simulink model "ModelCurrentState"  (R2024b)
settings: Solver=VariableStepAuto  StartTime=0.0  StopTime=StopTime  MaxStep=0.001  RelTol=1e-3
model workspace: external: MAT-File 3DModelInputs.mat (data not in the file)
undefined symbols (not defined in the file): GripStrength, KillswitchFinalValue, KillswitchInitialValue, KillswitchStepTime, LeftLowerArmLength, PlaneTilt, RightLowerArmLength, UpperTorsoLength, X, Y, Z
libraries: nesl_utility x408, sm_lib x139, matrix_library x11, simulink x1
(part 12 of 14)

== matlab function ModelCurrentState/LW Input Function/Left Wrist Torque ==
  data: Time input; Killswitch input; JointTorqueLWX output; LWInputXA parameter; LWInputYA parameter; LWInputXB parameter; LWInputYB parameter; LWPositionSetpointX parameter; GlobalGain parameter; JointTorqueLWY output; LWConstantX parameter; LWConstantY parameter; LWTimeGainX parameter; LWTimeGainY parameter; LWInputXC parameter; LWInputYC parameter; LWPositionGainX parameter; LWPositionGainY parameter; TargetLWPositionX parameter; ModelingMode parameter; GlobalPCGain parameter; GlobalVCGain parameter; DampeningGlobalGain parameter; TargetImpactTime parameter; KinematicMode parameter; LWPositionSetpointY parameter; LWStartPositionX parameter; LWStartPositionY parameter; LWStartVelocityX parameter; LWStartVelocityY parameter; LWVCGainX parameter; LWVCGainY parameter; LWPCGainX parameter; LWPCGainY parameter; LWPositionInputX output; LWPositionInputY output; LWVelocityInputX output; LWVelocityInputY output; LWAccelerationInputX output; LWAccelerationInputY output; ZVCFLWTorqueX parameter; ZVCFLWTorqueY parameter; LWAoX parameter; LWAoY parameter; LWDampeningX parameter; LWDampeningY parameter; TargetLWPositionY parameter; TargetLWVelocityX parameter; TargetLWVelocityY parameter; LWPositionX input; LWPositionY input; LWVelocityX input; LWVelocityY input; LWAfX parameter; LWAfY parameter; LWInputXD parameter; LWInputXE parameter; LWInputXF parameter; LWInputXG parameter; LWInputYD parameter; LWInputYE parameter; LWInputYF parameter; LWInputYG parameter; LWLocaltoGlobalR input; LWTorqueGlobal input; LWJointTorqueInputGlobal output; LWConstraintTorque output
function [JointTorqueLWX,JointTorqueLWY,LWPositionInputX, LWPositionInputY,...
    LWVelocityInputX,LWVelocityInputY,LWAccelerationInputX,LWAccelerationInputY,...
    LWJointTorqueInputGlobal,LWConstraintTorque]...
    = fcn(Time,Killswitch, LWInputXA,LWInputYA, LWInputXB,LWInputYB, LWPositionSetpointX,GlobalGain,...
    LWConstantX, LWConstantY, LWTimeGainX, LWTimeGainY,...
    LWInputXC, LWInputYC, LWPositionGainX, LWPositionGainY,...
    TargetLWPositionX, ModelingMode,GlobalPCGain, GlobalVCGain,DampeningGlobalGain,TargetImpactTime,KinematicMode, LWPositionSetpointY, LWStartPositionX,...
    LWStartPositionY, LWStartVelocityX, LWStartVelocityY, LWVCGainX,...
    LWVCGainY, LWPCGainX, LWPCGainY, ZVCFLWTorqueX, ZVCFLWTorqueY, LWAoX,...
    LWAoY, LWDampeningX, LWDampeningY, TargetLWPositionY, TargetLWVelocityX,...
    TargetLWVelocityY, LWPositionX, LWPositionY, LWVelocityX, LWVelocityY,...
    LWAfX, LWAfY,LWInputXD, LWInputXE, LWInputXF, LWInputXG, LWInputYD, LWInputYE, LWInputYF, LWInputYG,LWLocaltoGlobalR,LWTorqueGlobal)

%Tau=Time/TargetImpactTime;
t=Time;

% %%%%%%%%%%%%%%%%%%%%%%%%%%%%%%%%%%%%%%%%%%%
% % Kinetic Input Selection and Calculation
% %%%%%%%%%%%%%%%%%%%%%%%%%%%%%%%%%%%%%%%%%%%

if ModelingMode==0
    % Values are all set to zero.
    JointTorqueLWX=0;
    JointTorqueLWY=0;
elseif ModelingMode==1
    % Control based strategy. Values are based on difference in value
    % between the current state and desired state.
    % LW Joint Rotational Deltas
    DeltaLWPositionX=LWPositionX-TargetLWPositionX;
    DeltaLWPositionY=LWPositionY-TargetLWPositionY;
    DeltaLWVelocityX=LWVelocityX-TargetLWVelocityX;
    DeltaLWVelocityY=LWVelocityY-TargetLWVelocityY;
    % Control Based Strategy
    JointTorqueLWX=DeltaLWPositionX*LWPCGainX*GlobalPCGain-DeltaLWVelocityX*LWVCGainX*GlobalVCGain-DampeningGlobalGain*LWDampeningX*LWVelocityX;
    JointTorqueLWY=DeltaLWPositionY*LWPCGainY*GlobalPCGain-DeltaLWVelocityY*LWVCGainY*GlobalVCGain-DampeningGlobalGain*LWDampeningY*LWVelocityY;
elseif ModelingMode==2
    % Forward Dynamics Based Strategy. Values are computed based on a
    % polynomial and a combination of dampening and position gained
    % factors.
    JointTorqueLWX=Killswitch*GlobalGain*(LWConstantX+LWTimeGainX*Time-LWPositionGainX*(LWPositionX-LWPositionSetpointX)...
    -LWDampeningX*LWVelocityX);
    JointTorqueLWY=Killswitch*GlobalGain*(LWConstantY+LWTimeGainY*Time-LWPositionGainY*(LWPositionY-LWPositionSetpointY)...
    -LWDampeningY*LWVelocityY);
elseif ModelingMode==3
    JointTorqueLWX=HexPolyInputFunction(LWInputXA,LWInputXB,LWInputXC,LWInputXD,LWInputXE,LWInputXF,LWInputXG,Time)*Killswitch;
    JointTorqueLWY=HexPolyInputFunction(LWInputYA,LWInputYB,LWInputYC,LWInputYD,LWInputYE,LWInputYF,LWInputYG,Time)*Killswitch;  
else
    %ZVCF Based Joint Torques. Values are pulled from model workspace and
    %held constant.
    JointTorqueLWX=ZVCFLWTorqueX;
    JointTorqueLWY=ZVCFLWTorqueY;
end

% Create a global vector of the joint torque inputs
LWJointTorqueInputLocal=cat(1,JointTorqueLWX,JointTorqueLWY,0);
LWJointTorqueInputGlobal=LWLocaltoGlobalR*LWJointTorqueInputLocal;
% 
% Compare total torque measured to input torques applied to see the
% constraint torque
LWConstraintTorque=LWTorqueGlobal-LWJointTorqueInputGlobal;

% %%%%%%%%%%%%%%%%%%%%%%%%%%%%%%%%%%%%%%%%%%%
% % Kinematic Input Selection and Calculation
% %%%%%%%%%%%%%%%%%%%%%%%%%%%%%%%%%%%%%%%%%%%

if KinematicMode==0
    % All kinematic values set to zero.
    LWPositionInputX=0;
    LWPositionInputY=0;
    LWVelocityInputX=0;
    LWVelocityInputY=0;
    LWAccelerationInputX=0;
    LWAccelerationInputY=0;
elseif KinematicMode==1
    % 1st Order Acceleration, 2nd Order Velocity, 3rd Order Position Solution
    PTX=TargetLWPositionX;       
    VTX=TargetLWVelocityX;
    PTY=TargetLWPositionY;
    VTY=TargetLWVelocityY;
    % Define Starting Position and Velocity
    PIX=LWStartPositionX;
    VIX=LWStartVelocityX;
    PIY=LWStartPositionY;
    VIY=LWStartVelocityY;
    AX=3*((VTX+VIX)*TargetImpactTime-2*(PTX-PIX))/TargetImpactTime^3;         % Constant in position equation
    BX=-2*((VTX+2*VIX)*TargetImpactTime-3*(PTX-PIX))/TargetImpactTime^2;         % Constant in position equation
    CX=VIX;         % Starting Velocity at Time Zero
    DX=PIX;         % Starting Position at Time Zero
    AY=3*((VTY+VIY)*TargetImpactTime-2*(PTY-PIY))/TargetImpactTime^3;         % Constant in position equation
    BY=-2*((VTY+2*VIY)*TargetImpactTime-3*(PTY-PIY))/TargetImpactTime^2;         % Constant in position equation
    CY=VIY;         % Starting Velocity at Time Zero
    DY=PIY;         % Starting Position at Time Zero
    % Equation for position as a function of time
    LWPositionInputX=AX*Time^3/3+BX*Time^2/2+CX*Time+DX;
    LWPositionInputY=AY*Time^3/3+BY*Time^2/2+CY*Time+DY;
    LWVelocityInputX=AX*Time^2+BX*Time+CX;
    LWVelocityInputY=AY*Time^2+BY*Time+CY;
    LWAccelerationInputX=2*AX*Time+BX;
    LWAccelerationInputY=2*AY*Time+BY;
elseif KinematicMode==2
    % 2nd Order Acceleration, 3rd Order Velocity, 4th Order Position Solution
    Tt=TargetImpactTime;
    t=Time;
    PoX=LWStartPositionX;
    PoY=LWStartPositionY;
    VoX=LWStartVelocityX;
    VoY=LWStartVelocityY;
    PfX=TargetLWPositionX;
    PfY=TargetLWPositionY;
    VfX=TargetLWVelocityX;
    VfY=TargetLWVelocityY;
    AoX=LWAoX;
    AoY=LWAoY;
    LWPositionInputX=PoX + VoX*t + (AoX*t^2)/2 - (t^3*(4*PoX - 4*PfX + Tt*VfX + 3*Tt*VoX + AoX*Tt^2))/Tt^3 + (t^4*(6*PoX - 6*PfX + 2*Tt*VfX + 4*Tt*VoX + AoX*Tt^2))/(2*Tt^4);
    LWPositionInputY=PoY + VoY*t + (AoY*t^2)/2 - (t^3*(4*PoY - 4*PfY + Tt*VfY + 3*Tt*VoY + AoY*Tt^2))/Tt^3 + (t^4*(6*PoY - 6*PfY + 2*Tt*VfY + 4*Tt*VoY + AoY*Tt^2))/(2*Tt^4);
    LWVelocityInputX=VoX + AoX*t - (3*t^2*(4*PoX - 4*PfX + Tt*VfX + 3*Tt*VoX + AoX*Tt^2))/Tt^3 + (2*t^3*(6*PoX - 6*PfX + 2*Tt*VfX + 4*Tt*VoX + AoX*Tt^2))/Tt^4;
    LWVelocityInputY=VoY + AoY*t - (3*t^2*(4*PoY - 4*PfY + Tt*VfY + 3*Tt*VoY + AoY*Tt^2))/Tt^3 + (2*t^3*(6*PoY - 6*PfY + 2*Tt*VfY + 4*Tt*VoY + AoY*Tt^2))/Tt^4;
    LWAccelerationInputX=AoX + (6*t^2*(6*PoX - 6*PfX + 2*Tt*VfX + 4*Tt*VoX + AoX*Tt^2))/Tt^4 - (6*t*(4*PoX - 4*PfX + Tt*VfX + 3*Tt*VoX + AoX*Tt^2))/Tt^3;
    LWAccelerationInputY=AoY + (6*t^2*(6*PoY - 6*PfY + 2*Tt*VfY + 4*Tt*VoY + AoY*Tt^2))/Tt^4 - (6*t*(4*PoY - 4*PfY + Tt*VfY + 3*Tt*VoY + AoY*Tt^2))/Tt^3;
else
    % 3rd Order Acceleration, 4th Order Velocity, 5th Order Position Solution
    Tt=TargetImpactTime;
    t=Time;
    PoX=LWStartPositionX;
    PoY=LWStartPositionY;
    VoX=LWStartVelocityX;
    VoY=LWStartVelocityY;
    PfX=TargetLWPositionX;
    PfY=TargetLWPositionY;
    VfX=TargetLWVelocityX;
    VfY=TargetLWVelocityY;
    AoX=LWAoX;
    AoY=LWAoY;
    AfX=LWAfX;
    AfY=LWAfY;
    LWPositionInputX=PoX+VoX*t+(AoX*t^2)/2-(t^5*(12*PoX-12*PfX+6*Tt*VfX+6*Tt*VoX-AfX*Tt^2+AoX*Tt^2))/(2*Tt^5)-(t^3*(20*PoX-20*PfX+8*Tt*VfX+12*Tt*VoX-AfX*Tt^2+3*AoX*Tt^2))/(2*Tt^3)+(t^4*(30*PoX-30*PfX+14*Tt*VfX+16*Tt*VoX-2*AfX*Tt^2+3*AoX*Tt^2))/(2*Tt^4);
    LWPositionInputY=PoY+VoY*t+(AoY*t^2)/2-(t^5*(12*PoY-12*PfY+6*Tt*VfY+6*Tt*VoY-AfY*Tt^2+AoY*Tt^2))/(2*Tt^5)-(t^3*(20*PoY-20*PfY+8*Tt*VfY+12*Tt*VoY-AfY*Tt^2+3*AoY*Tt^2))/(2*Tt^3)+(t^4*(30*PoY-30*PfY+14*Tt*VfY+16*Tt*VoY-2*AfY*Tt^2+3*AoY*Tt^2))/(2*Tt^4);  
    LWVelocityInputX=VoX+AoX*t-(5*t^4*(12*PoX-12*PfX+6*Tt*VfX+6*Tt*VoX-AfX*Tt^2+AoX*Tt^2))/(2*Tt^5)-(3*t^2*(20*PoX-20*PfX+8*Tt*VfX+12*Tt*VoX-AfX*Tt^2+3*AoX*Tt^2))/(2*Tt^3)+(2*t^3*(30*PoX-30*PfX+14*Tt*VfX+16*Tt*VoX-2*AfX*Tt^2+3*AoX*Tt^2))/Tt^4;
    LWVelocityInputY=VoY+AoY*t-(5*t^4*(12*PoY-12*PfY+6*Tt*VfY+6*Tt*VoY-AfY*Tt^2+AoY*Tt^2))/(2*Tt^5)-(3*t^2*(20*PoY-20*PfY+8*Tt*VfY+12*Tt*VoY-AfY*Tt^2+3*AoY*Tt^2))/(2*Tt^3)+(2*t^3*(30*PoY-30*PfY+14*Tt*VfY+16*Tt*VoY-2*AfY*Tt^2+3*AoY*Tt^2))/Tt^4;
    LWAccelerationInputX=AoX-(3*t*(20*PoX-20*PfX+8*Tt*VfX+12*Tt*VoX-AfX*Tt^2+3*AoX*Tt^2))/Tt^3-(10*t^3*(12*PoX-12*PfX+6*Tt*VfX+6*Tt*VoX-AfX*Tt^2+AoX*Tt^2))/Tt^5+(6*t^2*(30*PoX-30*PfX+14*Tt*VfX+16*Tt*VoX-2*AfX*Tt^2+3*AoX*Tt^2))/Tt^4;
    LWAccelerationInputY=AoY-(3*t*(20*PoY-20*PfY+8*Tt*VfY+12*Tt*VoY-AfY*Tt^2+3*AoY*Tt^2))/Tt^3-(10*t^3*(12*PoY-12*PfY+6*Tt*VfY+6*Tt*VoY-AfY*Tt^2+AoY*Tt^2))/Tt^5+(6*t^2*(30*PoY-30*PfY+14*Tt*VfY+16*Tt*VoY-2*AfY*Tt^2+3*AoY*Tt^2))/Tt^4;
end


% Calculate Higher Order Derivatives of the Position Outputs
LWJerkX=gradient(LWAccelerationInputX,t);
LWJerkY=gradient(LWAccelerationInputY,t);
LWSnapX=gradient(LWJerkX,t);
LWSnapY=gradient(LWJerkY,t);
LWCrackleX=gradient(LWSnapX,t);
LWCrackleY=gradient(LWSnapY,t);
LWPopX=gradient(LWCrackleX,t);
LWPopY=gradient(LWCrackleY,t);

== matlab function ModelCurrentState/RW Input Function/Right Wrist Torque ==
  data: Time input; Killswitch input; JointTorqueRWX output; RWInputXA parameter; RWInputYA parameter; RWInputXB parameter; RWInputYB parameter; RWPositionSetpointX parameter; GlobalGain parameter; JointTorqueRWY output; RWConstantX parameter; RWConstantY parameter; RWTimeGainX parameter; RWTimeGainY parameter; RWInputXC parameter; RWInputYC parameter; RWPositionGainX parameter; RWPositionGainY parameter; TargetRWPositionX parameter; ModelingMode parameter; GlobalPCGain parameter; GlobalVCGain parameter; DampeningGlobalGain parameter; TargetImpactTime parameter; KinematicMode parameter; RWVCGainY parameter; RWPCGainX parameter; RWPCGainY parameter; ZVCFRWTorqueX parameter; ZVCFRWTorqueY parameter; TargetRWPositionY parameter; TargetRWVelocityX parameter; TargetRWVelocityY parameter; RWAoX parameter; RWPositionInputX output; RWPositionInputY output; RWVelocityInputX output; RWVelocityInputY output; RWAccelerationInputX output; RWAccelerationInputY output; RWAoY parameter; RWDampeningX parameter; RWDampeningY parameter; RWPositionX input; RWPositionY input; RWStartPositionX parameter; RWStartPositionY parameter; RWStartVelocityX parameter; RWStartVelocityY parameter; RWVCGainX parameter; RWPositionSetpointY parameter; RWVelocityX input; RWVelocityY input; RWAfX parameter; RWAfY parameter; RWInputXD parameter; RWInputXE parameter; RWInputXF parameter; RWInputXG parameter; RWInputYD parameter; RWInputYE parameter; RWInputYF parameter; RWInputYG parameter; RWLocaltoGlobalR input; RWTorqueGlobal input; RWJointTorqueInputGlobal output; RWConstraintTorque output
function [JointTorqueRWX,JointTorqueRWY,RWPositionInputX, RWPositionInputY,...
    RWVelocityInputX,RWVelocityInputY,RWAccelerationInputX,RWAccelerationInputY,...
    RWJointTorqueInputGlobal,RWConstraintTorque]...
    = fcn(Time,Killswitch, RWInputXA,RWInputYA, RWInputXB,RWInputYB, RWPositionSetpointX,GlobalGain,...
    RWConstantX, RWConstantY, RWTimeGainX, RWTimeGainY,...
    RWInputXC, RWInputYC, RWPositionGainX, RWPositionGainY,...
    TargetRWPositionX, ModelingMode,GlobalPCGain, GlobalVCGain,...
    DampeningGlobalGain,TargetImpactTime,KinematicMode, RWVCGainY,...
    RWPCGainX, RWPCGainY, ZVCFRWTorqueX, ...
    ZVCFRWTorqueY, TargetRWPositionY, TargetRWVelocityX, TargetRWVelocityY,...
    RWAoX, RWAoY, RWDampeningX, RWDampeningY, RWPositionX, RWPositionY, RWStartPositionX,...
    RWStartPositionY, RWStartVelocityX, RWStartVelocityY, RWVCGainX,...
    RWPositionSetpointY, RWVelocityX, RWVelocityY,RWAfX, RWAfY,RWInputXD, RWInputXE, RWInputXF,...
RWInputXG, RWInputYD, RWInputYE, RWInputYF, RWInputYG,RWLocaltoGlobalR,RWTorqueGlobal)

%Tau=Time/TargetImpactTime;
t=Time;

% %%%%%%%%%%%%%%%%%%%%%%%%%%%%%%%%%%%%%%%%%%%
% % Kinetic Input Selection and Calculation
% %%%%%%%%%%%%%%%%%%%%%%%%%%%%%%%%%%%%%%%%%%%

if ModelingMode==0
    % Values are all set to zero.
    JointTorqueRWX=0;
    JointTorqueRWY=0;
elseif ModelingMode==1
    % Control based strategy. Values are based on difference in value
    % between the current state and desired state.
    % RW Joint Rotational Deltas
    DeltaRWPositionX=RWPositionX-TargetRWPositionX;
    DeltaRWPositionY=RWPositionY-TargetRWPositionY;
    DeltaRWVelocityX=RWVelocityX-TargetRWVelocityX;
    DeltaRWVelocityY=RWVelocityY-TargetRWVelocityY;
    % Control Based Strategy
    JointTorqueRWX=DeltaRWPositionX*RWPCGainX*GlobalPCGain-DeltaRWVelocityX*RWVCGainX*GlobalVCGain-DampeningGlobalGain*RWDampeningX*RWVelocityX;
    JointTorqueRWY=DeltaRWPositionY*RWPCGainY*GlobalPCGain-DeltaRWVelocityY*RWVCGainY*GlobalVCGain-DampeningGlobalGain*RWDampeningY*RWVelocityY;
elseif ModelingMode==2
    % Forward Dynamics Based Strategy. Values are computed based on a
    % polynomial and a combination of dampening and position gained
    % factors.
    JointTorqueRWX=Killswitch*GlobalGain*(RWConstantX+RWTimeGainX*Time-RWPositionGainX*(RWPositionX-RWPositionSetpointX)...
    -RWDampeningX*RWVelocityX);
    JointTorqueRWY=Killswitch*GlobalGain*(RWConstantY+RWTimeGainY*Time-RWPositionGainY*(RWPositionY-RWPositionSetpointY)...
    -RWDampeningY*RWVelocityY);
elseif ModelingMode==3
    JointTorqueRWX=HexPolyInputFunction(RWInputXA,RWInputXB,RWInputXC,RWInputXD,RWInputXE,RWInputXF,RWInputXG,Time)*Killswitch;
    JointTorqueRWY=HexPolyInputFunction(RWInputYA,RWInputYB,RWInputYC,RWInputYD,RWInputYE,RWInputYF,RWInputYG,Time)*Killswitch;  
else
    %ZVCF Based Joint Torques. Values are pulled from model workspace and
    %held constant.
    JointTorqueRWX=ZVCFRWTorqueX;
    JointTorqueRWY=ZVCFRWTorqueY;
end

% Create a global vector of the joint torque inputs
RWJointTorqueInputLocal=cat(1,JointTorqueRWX,JointTorqueRWY,0);
RWJointTorqueInputGlobal=RWLocaltoGlobalR*RWJointTorqueInputLocal;

% Compare total torque measured to input torques applied to see the
% constraint torque

RWConstraintTorque=RWTorqueGlobal-RWJointTorqueInputGlobal;

% %%%%%%%%%%%%%%%%%%%%%%%%%%%%%%%%%%%%%%%%%%%
% % Kinematic Input Selection and Calculation
% %%%%%%%%%%%%%%%%%%%%%%%%%%%%%%%%%%%%%%%%%%%

if KinematicMode==0
    % All kinematic values set to zero.
    RWPositionInputX=0;
    RWPositionInputY=0;
    RWVelocityInputX=0;
    RWVelocityInputY=0;
    RWAccelerationInputX=0;
    RWAccelerationInputY=0;
elseif KinematicMode==1
    % 1st Order Acceleration, 2nd Order Velocity, 3rd Order Position Solution
    PTX=TargetRWPositionX;       
    VTX=TargetRWVelocityX;
    PTY=TargetRWPositionY;
    VTY=TargetRWVelocityY;
    % Define Starting Position and Velocity
    PIX=RWStartPositionX;
    VIX=RWStartVelocityX;
    PIY=RWStartPositionY;
    VIY=RWStartVelocityY;
    AX=3*((VTX+VIX)*TargetImpactTime-2*(PTX-PIX))/TargetImpactTime^3;         % Constant in position equation
    BX=-2*((VTX+2*VIX)*TargetImpactTime-3*(PTX-PIX))/TargetImpactTime^2;         % Constant in position equation
    CX=VIX;         % Starting Velocity at Time Zero
    DX=PIX;         % Starting Position at Time Zero
    AY=3*((VTY+VIY)*TargetImpactTime-2*(PTY-PIY))/TargetImpactTime^3;         % Constant in position equation
    BY=-2*((VTY+2*VIY)*TargetImpactTime-3*(PTY-PIY))/TargetImpactTime^2;         % Constant in position equation
    CY=VIY;         % Starting Velocity at Time Zero
    DY=PIY;         % Starting Position at Time Zero
    % Equation for position as a function of time
    RWPositionInputX=AX*Time^3/3+BX*Time^2/2+CX*Time+DX;
    RWPositionInputY=AY*Time^3/3+BY*Time^2/2+CY*Time+DY;
    RWVelocityInputX=AX*Time^2+BX*Time+CX;
    RWVelocityInputY=AY*Time^2+BY*Time+CY;
    RWAccelerationInputX=2*AX*Time+BX;
    RWAccelerationInputY=2*AY*Time+BY;
elseif KinematicMode==2
    % 2nd Order Acceleration, 3rd Order Velocity, 4th Order Position Solution
    Tt=TargetImpactTime;
    t=Time;
    PoX=RWStartPositionX;
    PoY=RWStartPositionY;
    VoX=RWStartVelocityX;
    VoY=RWStartVelocityY;
    PfX=TargetRWPositionX;
    PfY=TargetRWPositionY;
    VfX=TargetRWVelocityX;
    VfY=TargetRWVelocityY;
    AoX=RWAoX;
    AoY=RWAoY;
    RWPositionInputX=PoX + VoX*t + (AoX*t^2)/2 - (t^3*(4*PoX - 4*PfX + Tt*VfX + 3*Tt*VoX + AoX*Tt^2))/Tt^3 + (t^4*(6*PoX - 6*PfX + 2*Tt*VfX + 4*Tt*VoX + AoX*Tt^2))/(2*Tt^4);
    RWPositionInputY=PoY + VoY*t + (AoY*t^2)/2 - (t^3*(4*PoY - 4*PfY + Tt*VfY + 3*Tt*VoY + AoY*Tt^2))/Tt^3 + (t^4*(6*PoY - 6*PfY + 2*Tt*VfY + 4*Tt*VoY + AoY*Tt^2))/(2*Tt^4);
    RWVelocityInputX=VoX + AoX*t - (3*t^2*(4*PoX - 4*PfX + Tt*VfX + 3*Tt*VoX + AoX*Tt^2))/Tt^3 + (2*t^3*(6*PoX - 6*PfX + 2*Tt*VfX + 4*Tt*VoX + AoX*Tt^2))/Tt^4;
    RWVelocityInputY=VoY + AoY*t - (3*t^2*(4*PoY - 4*PfY + Tt*VfY + 3*Tt*VoY + AoY*Tt^2))/Tt^3 + (2*t^3*(6*PoY - 6*PfY + 2*Tt*VfY + 4*Tt*VoY + AoY*Tt^2))/Tt^4;
    RWAccelerationInputX=AoX + (6*t^2*(6*PoX - 6*PfX + 2*Tt*VfX + 4*Tt*VoX + AoX*Tt^2))/Tt^4 - (6*t*(4*PoX - 4*PfX + Tt*VfX + 3*Tt*VoX + AoX*Tt^2))/Tt^3;
    RWAccelerationInputY=AoY + (6*t^2*(6*PoY - 6*PfY + 2*Tt*VfY + 4*Tt*VoY + AoY*Tt^2))/Tt^4 - (6*t*(4*PoY - 4*PfY + Tt*VfY + 3*Tt*VoY + AoY*Tt^2))/Tt^3;
else
    % 3rd Order Acceleration, 4th Order Velocity, 5th Order Position Solution
    Tt=TargetImpactTime;
    t=Time;
    PoX=RWStartPositionX;
    PoY=RWStartPositionY;
    VoX=RWStartVelocityX;
    VoY=RWStartVelocityY;
    PfX=TargetRWPositionX;
    PfY=TargetRWPositionY;
    VfX=TargetRWVelocityX;
    VfY=TargetRWVelocityY;
    AoX=RWAoX;
    AoY=RWAoY;
    AfX=RWAfX;
    AfY=RWAfY;
    RWPositionInputX=PoX+VoX*t+(AoX*t^2)/2-(t^5*(12*PoX-12*PfX+6*Tt*VfX+6*Tt*VoX-AfX*Tt^2+AoX*Tt^2))/(2*Tt^5)-(t^3*(20*PoX-20*PfX+8*Tt*VfX+12*Tt*VoX-AfX*Tt^2+3*AoX*Tt^2))/(2*Tt^3)+(t^4*(30*PoX-30*PfX+14*Tt*VfX+16*Tt*VoX-2*AfX*Tt^2+3*AoX*Tt^2))/(2*Tt^4);
    RWPositionInputY=PoY+VoY*t+(AoY*t^2)/2-(t^5*(12*PoY-12*PfY+6*Tt*VfY+6*Tt*VoY-AfY*Tt^2+AoY*Tt^2))/(2*Tt^5)-(t^3*(20*PoY-20*PfY+8*Tt*VfY+12*Tt*VoY-AfY*Tt^2+3*AoY*Tt^2))/(2*Tt^3)+(t^4*(30*PoY-30*PfY+14*Tt*VfY+16*Tt*VoY-2*AfY*Tt^2+3*AoY*Tt^2))/(2*Tt^4);  
    RWVelocityInputX=VoX+AoX*t-(5*t^4*(12*PoX-12*PfX+6*Tt*VfX+6*Tt*VoX-AfX*Tt^2+AoX*Tt^2))/(2*Tt^5)-(3*t^2*(20*PoX-20*PfX+8*Tt*VfX+12*Tt*VoX-AfX*Tt^2+3*AoX*Tt^2))/(2*Tt^3)+(2*t^3*(30*PoX-30*PfX+14*Tt*VfX+16*Tt*VoX-2*AfX*Tt^2+3*AoX*Tt^2))/Tt^4;
    RWVelocityInputY=VoY+AoY*t-(5*t^4*(12*PoY-12*PfY+6*Tt*VfY+6*Tt*VoY-AfY*Tt^2+AoY*Tt^2))/(2*Tt^5)-(3*t^2*(20*PoY-20*PfY+8*Tt*VfY+12*Tt*VoY-AfY*Tt^2+3*AoY*Tt^2))/(2*Tt^3)+(2*t^3*(30*PoY-30*PfY+14*Tt*VfY+16*Tt*VoY-2*AfY*Tt^2+3*AoY*Tt^2))/Tt^4;
    RWAccelerationInputX=AoX-(3*t*(20*PoX-20*PfX+8*Tt*VfX+12*Tt*VoX-AfX*Tt^2+3*AoX*Tt^2))/Tt^3-(10*t^3*(12*PoX-12*PfX+6*Tt*VfX+6*Tt*VoX-AfX*Tt^2+AoX*Tt^2))/Tt^5+(6*t^2*(30*PoX-30*PfX+14*Tt*VfX+16*Tt*VoX-2*AfX*Tt^2+3*AoX*Tt^2))/Tt^4;
    RWAccelerationInputY=AoY-(3*t*(20*PoY-20*PfY+8*Tt*VfY+12*Tt*VoY-AfY*Tt^2+3*AoY*Tt^2))/Tt^3-(10*t^3*(12*PoY-12*PfY+6*Tt*VfY+6*Tt*VoY-AfY*Tt^2+AoY*Tt^2))/Tt^5+(6*t^2*(30*PoY-30*PfY+14*Tt*VfY+16*Tt*VoY-2*AfY*Tt^2+3*AoY*Tt^2))/Tt^4;
end

% Calculate Higher Order Derivatives of the Position Outputs
RWJerkX=gradient(RWAccelerationInputX,t);
RWJerkY=gradient(RWAccelerationInputY,t);
RWSnapX=gradient(RWJerkX,t);
RWSnapY=gradient(RWJerkY,t);
RWCrackleX=gradient(RWSnapX,t);
RWCrackleY=gradient(RWSnapY,t);
RWPopX=gradient(RWCrackleX,t);
RWPopY=gradient(RWCrackleY,t);

== matlab function ModelCurrentState/LE Input Function/Left Elbow Input Torque ==
  data: Time input; Killswitch input; JointTorqueLE output; LEPositionInput output; LEInputB parameter; LEPositionSetpoint parameter; GlobalGain parameter; LEDampening parameter; ModelingMode parameter; GlobalPCGain parameter; GlobalVCGain parameter; DampeningGlobalGain parameter; TargetImpactTime parameter; KinematicMode parameter; LEAo parameter; LEStartPosition parameter; LEStartVelocity parameter; LEVCGain parameter; TargetLEVelocity parameter; TargetLEPosition parameter; LEPositionGain parameter; LEInputC parameter; LETimeGain parameter; LEVelocityInput output; LEAccelerationInput output; LEConstant parameter; LEPosition input; LEVelocity input; ZVCFLETorque parameter; LEPCGain parameter; LEInputA parameter; LEAf parameter; LEInputD parameter; LEInputE parameter; LEInputF parameter; LEInputG parameter
function [JointTorqueLE,LEPositionInput,LEVelocityInput,...
    LEAccelerationInput]  = fcn(Time,Killswitch,...
    LEInputB,LEPositionSetpoint,GlobalGain,...
    LEDampening, ModelingMode,GlobalPCGain, GlobalVCGain,...
    DampeningGlobalGain,TargetImpactTime,KinematicMode, LEAo,LEStartPosition,...
    LEStartVelocity,LEVCGain,...
    TargetLEVelocity,TargetLEPosition, ...
    LEPositionGain,LEInputC,...
    LETimeGain, LEConstant, LEPosition,LEVelocity, ZVCFLETorque, LEPCGain, LEInputA,...
    LEAf, LEInputD, LEInputE, LEInputF, LEInputG)

%Tau=Time/TargetImpactTime;
t=Time;

% %%%%%%%%%%%%%%%%%%%%%%%%%%%%%%%%%%%%%%%%%%%
% % Kinetic Input Selection and Calculation
% %%%%%%%%%%%%%%%%%%%%%%%%%%%%%%%%%%%%%%%%%%%

if ModelingMode==0
    % Values are all set to zero.
    JointTorqueLE=0;
elseif ModelingMode==1
    % Control based strategy. Values are based on difference in value
    % between the current state and desired state.
    % LE Joint Rotational Deltas
    DeltaLEPosition=LEPosition-TargetLEPosition;
    DeltaLEVelocity=LEVelocity-TargetLEVelocity;
    % Control Based Strategy
    JointTorqueLE=DeltaLEPosition*LEPCGain*GlobalPCGain-DeltaLEVelocity*LEVCGain*GlobalVCGain-DampeningGlobalGain*LEDampening*LEVelocity;
elseif ModelingMode==2
    % Forward Dynamics Based Strategy. Values are computed based on a
    % polynomial and a combination of dampening and position gained
    % factors.
    JointTorqueLE=Killswitch*GlobalGain*(LEConstant+LETimeGain*Time-LEPositionGain*(LEPosition-LEPositionSetpoint)...
    -LEDampening*LEVelocity);
elseif ModelingMode==3
    JointTorqueLE=HexPolyInputFunction(LEInputA,LEInputB,LEInputC,LEInputD,LEInputE,LEInputF,LEInputG,Time)*Killswitch;
else
    %ZVCF Based Joint Torques. Values are pulled from model workspace and
    %held constant.
    JointTorqueLE=ZVCFLETorque;
end

% %%%%%%%%%%%%%%%%%%%%%%%%%%%%%%%%%%%%%%%%%%%
% % Kinematic Input Selection and Calculation
% %%%%%%%%%%%%%%%%%%%%%%%%%%%%%%%%%%%%%%%%%%%

if KinematicMode==0
    % All kinematic values set to zero.
    LEPositionInput=0;
    LEPositionInputY=0;
    LEVelocityInput=0;
    LEVelocityInputY=0;
    LEAccelerationInput=0;
    LEAccelerationInputY=0;
elseif KinematicMode==1
    % 1st Order Acceleration, 2nd Order Velocity, 3rd Order Position Solution
    PTX=TargetLEPosition;       
    VTX=TargetLEVelocity;
    % Define Starting Position and Velocity
    PIX=LEStartPosition;
    VIX=LEStartVelocity;
    AX=3*((VTX+VIX)*TargetImpactTime-2*(PTX-PIX))/TargetImpactTime^3;         % Constant in position equation
    BX=-2*((VTX+2*VIX)*TargetImpactTime-3*(PTX-PIX))/TargetImpactTime^2;         % Constant in position equation
    CX=VIX;         % Starting Velocity at Time Zero
    DX=PIX;         % Starting Position at Time Zero
    % Equation for position as a function of time
    LEPositionInput=AX*Time^3/3+BX*Time^2/2+CX*Time+DX;
    LEVelocityInput=AX*Time^2+BX*Time+CX;
    LEAccelerationInput=2*AX*Time+BX;
elseif KinematicMode==2
    % 2nd Order Acceleration, 3rd Order Velocity, 4th Order Position Solution
    Tt=TargetImpactTime;
    t=Time;
    PoX=LEStartPosition;
    VoX=LEStartVelocity;
    PfX=TargetLEPosition;
    VfX=TargetLEVelocity;
    AoX=LEAo;
    LEPositionInput=PoX + VoX*t + (AoX*t^2)/2 - (t^3*(4*PoX - 4*PfX + Tt*VfX + 3*Tt*VoX + AoX*Tt^2))/Tt^3 + (t^4*(6*PoX - 6*PfX + 2*Tt*VfX + 4*Tt*VoX + AoX*Tt^2))/(2*Tt^4);
    LEVelocityInput=VoX + AoX*t - (3*t^2*(4*PoX - 4*PfX + Tt*VfX + 3*Tt*VoX + AoX*Tt^2))/Tt^3 + (2*t^3*(6*PoX - 6*PfX + 2*Tt*VfX + 4*Tt*VoX + AoX*Tt^2))/Tt^4;
    LEAccelerationInput=AoX + (6*t^2*(6*PoX - 6*PfX + 2*Tt*VfX + 4*Tt*VoX + AoX*Tt^2))/Tt^4 - (6*t*(4*PoX - 4*PfX + Tt*VfX + 3*Tt*VoX + AoX*Tt^2))/Tt^3;
else
    % 3rd Order Acceleration, 4th Order Velocity, 5th Order Position Solution
    Tt=TargetImpactTime;
    t=Time;
    PoX=LEStartPosition;
    VoX=LEStartVelocity;
    PfX=TargetLEPosition;
    VfX=TargetLEVelocity;
    AoX=LEAo;
    AfX=LEAf;
    LEPositionInput=PoX+VoX*t+(AoX*t^2)/2-(t^5*(12*PoX-12*PfX+6*Tt*VfX+6*Tt*VoX-AfX*Tt^2+AoX*Tt^2))/(2*Tt^5)-(t^3*(20*PoX-20*PfX+8*Tt*VfX+12*Tt*VoX-AfX*Tt^2+3*AoX*Tt^2))/(2*Tt^3)+(t^4*(30*PoX-30*PfX+14*Tt*VfX+16*Tt*VoX-2*AfX*Tt^2+3*AoX*Tt^2))/(2*Tt^4);
    LEVelocityInput=VoX+AoX*t-(5*t^4*(12*PoX-12*PfX+6*Tt*VfX+6*Tt*VoX-AfX*Tt^2+AoX*Tt^2))/(2*Tt^5)-(3*t^2*(20*PoX-20*PfX+8*Tt*VfX+12*Tt*VoX-AfX*Tt^2+3*AoX*Tt^2))/(2*Tt^3)+(2*t^3*(30*PoX-30*PfX+14*Tt*VfX+16*Tt*VoX-2*AfX*Tt^2+3*AoX*Tt^2))/Tt^4;
    LEAccelerationInput=AoX-(3*t*(20*PoX-20*PfX+8*Tt*VfX+12*Tt*VoX-AfX*Tt^2+3*AoX*Tt^2))/Tt^3-(10*t^3*(12*PoX-12*PfX+6*Tt*VfX+6*Tt*VoX-AfX*Tt^2+AoX*Tt^2))/Tt^5+(6*t^2*(30*PoX-30*PfX+14*Tt*VfX+16*Tt*VoX-2*AfX*Tt^2+3*AoX*Tt^2))/Tt^4;
end

% Calculate Higher Order Derivatives of the Position Outputs
LEJerk=gradient(LEAccelerationInput,t);
LESnap=gradient(LEJerk,t);
LECrackle=gradient(LESnap,t);
LEPop=gradient(LECrackle,t);

== matlab function ModelCurrentState/RE Input Function/Right Elbow Input Torque ==
  data: Time input; Killswitch input; JointTorqueRE output; REPositionInput output; REInputB parameter; REPositionSetpoint parameter; GlobalGain parameter; REDampening parameter; ModelingMode parameter; GlobalPCGain parameter; GlobalVCGain parameter; DampeningGlobalGain parameter; TargetImpactTime parameter; KinematicMode parameter; REAo parameter; REStartPosition parameter; REStartVelocity parameter; REVCGain parameter; TargetREVelocity parameter; TargetREPosition parameter; REPositionGain parameter; REInputC parameter; RETimeGain parameter; REVelocityInput output; REAccelerationInput output; REConstant parameter; REPosition input; REVelocity input; ZVCFRETorque parameter; REPCGain parameter; REInputA parameter; REAf parameter; REInputD parameter; REInputE parameter; REInputF parameter; REInputG parameter
function [JointTorqueRE,REPositionInput,REVelocityInput,...
    REAccelerationInput]  = fcn(Time,Killswitch,...
    REInputB,REPositionSetpoint,GlobalGain,...
    REDampening, ModelingMode,GlobalPCGain, GlobalVCGain,...
    DampeningGlobalGain,TargetImpactTime,KinematicMode, REAo,REStartPosition,...
    REStartVelocity,REVCGain,...
    TargetREVelocity,TargetREPosition, ...
    REPositionGain,REInputC,...
    RETimeGain, REConstant, REPosition,REVelocity, ZVCFRETorque, REPCGain,...
    REInputA,REAf,REInputD, REInputE, REInputF, REInputG)

%Tau=Time/TargetImpactTime;
t=Time;

% %%%%%%%%%%%%%%%%%%%%%%%%%%%%%%%%%%%%%%%%%%%
% % Kinetic Input Selection and Calculation
% %%%%%%%%%%%%%%%%%%%%%%%%%%%%%%%%%%%%%%%%%%%

if ModelingMode==0
    % Values are all set to zero.
    JointTorqueRE=0;
elseif ModelingMode==1
    % Control based strategy. Values are based on difference in value
    % between the current state and desired state.
    % RE Joint Rotational Deltas
    DeltaREPosition=REPosition-TargetREPosition;
    DeltaREVelocity=REVelocity-TargetREVelocity;
    % Control Based Strategy
    JointTorqueRE=DeltaREPosition*REPCGain*GlobalPCGain-DeltaREVelocity*REVCGain*GlobalVCGain-DampeningGlobalGain*REDampening*REVelocity;
elseif ModelingMode==2
    % Forward Dynamics Based Strategy. Values are computed based on a
    % polynomial and a combination of dampening and position gained
    % factors.
    JointTorqueRE=Killswitch*GlobalGain*(REConstant+RETimeGain*Time-REPositionGain*(REPosition-REPositionSetpoint)...
    -REDampening*REVelocity);
elseif ModelingMode==3
    JointTorqueRE=HexPolyInputFunction(REInputA,REInputB,REInputC,REInputD,REInputE,REInputF,REInputG,Time)*Killswitch;
else
    %ZVCF Based Joint Torques. Values are pulled from model workspace and
    %held constant.
    JointTorqueRE=ZVCFRETorque;
end

% %%%%%%%%%%%%%%%%%%%%%%%%%%%%%%%%%%%%%%%%%%%
% % Kinematic Input Selection and Calculation
% %%%%%%%%%%%%%%%%%%%%%%%%%%%%%%%%%%%%%%%%%%%

% Manual Set Option
% KinematicMode=3;

if KinematicMode==0
    % All kinematic values set to zero.
    REPositionInput=0;
    REVelocityInput=0;
    REAccelerationInput=0;
elseif KinematicMode==1
    % 1st Order Acceleration, 2nd Order Velocity, 3rd Order Position Solution
    PTX=TargetREPosition;       
    VTX=TargetREVelocity;
    % Define Starting Position and Velocity
    PIX=REStartPosition;
    VIX=REStartVelocity;
    AX=3*((VTX+VIX)*TargetImpactTime-2*(PTX-PIX))/TargetImpactTime^3;         % Constant in position equation
    BX=-2*((VTX+2*VIX)*TargetImpactTime-3*(PTX-PIX))/TargetImpactTime^2;         % Constant in position equation
    CX=VIX;         % Starting Velocity at Time Zero
    DX=PIX;         % Starting Position at Time Zero
    % Equation for position as a function of time
    REPositionInput=AX*Time^3/3+BX*Time^2/2+CX*Time+DX;
    REVelocityInput=AX*Time^2+BX*Time+CX;
    REAccelerationInput=2*AX*Time+BX;
elseif KinematicMode==2
    % 2nd Order Acceleration, 3rd Order Velocity, 4th Order Position Solution
    Tt=TargetImpactTime;
    t=Time;
    PoX=REStartPosition;
    VoX=REStartVelocity;
    PfX=TargetREPosition;
    VfX=TargetREVelocity;
    AoX=REAo;
    REPositionInput=PoX + VoX*t + (AoX*t^2)/2 - (t^3*(4*PoX - 4*PfX + Tt*VfX + 3*Tt*VoX + AoX*Tt^2))/Tt^3 + (t^4*(6*PoX - 6*PfX + 2*Tt*VfX + 4*Tt*VoX + AoX*Tt^2))/(2*Tt^4);
    REVelocityInput=VoX + AoX*t - (3*t^2*(4*PoX - 4*PfX + Tt*VfX + 3*Tt*VoX + AoX*Tt^2))/Tt^3 + (2*t^3*(6*PoX - 6*PfX + 2*Tt*VfX + 4*Tt*VoX + AoX*Tt^2))/Tt^4;
    REAccelerationInput=AoX + (6*t^2*(6*PoX - 6*PfX + 2*Tt*VfX + 4*Tt*VoX + AoX*Tt^2))/Tt^4 - (6*t*(4*PoX - 4*PfX + Tt*VfX + 3*Tt*VoX + AoX*Tt^2))/Tt^3;
else
    % 3rd Order Acceleration, 4th Order Velocity, 5th Order Position Solution
    Tt=TargetImpactTime;
    t=Time;
    PoX=REStartPosition;
    VoX=REStartVelocity;
    PfX=TargetREPosition;
    VfX=TargetREVelocity;
    AoX=REAo;
    AfX=REAf;
    REPositionInput=PoX+VoX*t+(AoX*t^2)/2-(t^5*(12*PoX-12*PfX+6*Tt*VfX+6*Tt*VoX-AfX*Tt^2+AoX*Tt^2))/(2*Tt^5)-(t^3*(20*PoX-20*PfX+8*Tt*VfX+12*Tt*VoX-AfX*Tt^2+3*AoX*Tt^2))/(2*Tt^3)+(t^4*(30*PoX-30*PfX+14*Tt*VfX+16*Tt*VoX-2*AfX*Tt^2+3*AoX*Tt^2))/(2*Tt^4);
    REVelocityInput=VoX+AoX*t-(5*t^4*(12*PoX-12*PfX+6*Tt*VfX+6*Tt*VoX-AfX*Tt^2+AoX*Tt^2))/(2*Tt^5)-(3*t^2*(20*PoX-20*PfX+8*Tt*VfX+12*Tt*VoX-AfX*Tt^2+3*AoX*Tt^2))/(2*Tt^3)+(2*t^3*(30*PoX-30*PfX+14*Tt*VfX+16*Tt*VoX-2*AfX*Tt^2+3*AoX*Tt^2))/Tt^4;
    REAccelerationInput=AoX-(3*t*(20*PoX-20*PfX+8*Tt*VfX+12*Tt*VoX-AfX*Tt^2+3*AoX*Tt^2))/Tt^3-(10*t^3*(12*PoX-12*PfX+6*Tt*VfX+6*Tt*VoX-AfX*Tt^2+AoX*Tt^2))/Tt^5+(6*t^2*(30*PoX-30*PfX+14*Tt*VfX+16*Tt*VoX-2*AfX*Tt^2+3*AoX*Tt^2))/Tt^4;
end

% Calculate Higher Order Derivatives of the Position Outputs
REJerk=gradient(REAccelerationInput,t);
RESnap=gradient(REJerk,t);
RECrackle=gradient(RESnap,t);
REPop=gradient(RECrackle,t);

== matlab function ModelCurrentState/Right Hand/RW Unit Vector ==
  data: RWv input; RWSpeed output; RWvx input; RWvy input; RWvz input; RWuvx output; RWuvy output; RWuvz output
function [RWSpeed,RWuvx,RWuvy,RWuvz]  = fcn(RWv,RWvx,RWvy,RWvz)

RWSpeed=norm(RWv);
RWuvx=RWvx/RWSpeed;
RWuvy=RWvy/RWSpeed;
RWuvz=RWvz/RWSpeed;

== matlab function ModelCurrentState/LF Input Function/LF Input Torque ==
  data: Time input; Killswitch input; JointTorqueLF output; LFPositionInput output; LFInputB parameter; LFPositionSetpoint parameter; GlobalGain parameter; LFDampening parameter; ModelingMode parameter; GlobalPCGain parameter; GlobalVCGain parameter; DampeningGlobalGain parameter; TargetImpactTime parameter; KinematicMode parameter; LFAo parameter; LFStartPosition parameter; LFStartVelocity parameter; LFVCGain parameter; TargetLFVelocity parameter; TargetLFPosition parameter; LFPositionGain parameter; LFInputC parameter; LFTimeGain parameter; LFVelocityInput output; LFAccelerationInput output; LFConstant parameter; LFPosition input; LFVelocity input; ZVCFLFTorque parameter; LFPCGain parameter; LFInputA parameter; LFAf parameter; LFInputD parameter; LFInputE parameter; LFInputF parameter; LFInputG parameter
function [JointTorqueLF,LFPositionInput,LFVelocityInput,...
    LFAccelerationInput]  = fcn(Time,Killswitch,...
    LFInputB,LFPositionSetpoint,GlobalGain,...
    LFDampening, ModelingMode,GlobalPCGain, GlobalVCGain,...
    DampeningGlobalGain,TargetImpactTime,KinematicMode, LFAo,LFStartPosition,...
    LFStartVelocity,LFVCGain,...
    TargetLFVelocity,TargetLFPosition, ...
    LFPositionGain,LFInputC,...
    LFTimeGain, LFConstant, LFPosition,LFVelocity, ZVCFLFTorque, LFPCGain,...
    LFInputA,LFAf, LFInputD, LFInputE, LFInputF, LFInputG)

%Tau=Time/TargetImpactTime;
t=Time;

% %%%%%%%%%%%%%%%%%%%%%%%%%%%%%%%%%%%%%%%%%%%
% % Kinetic Input Selection and Calculation
% %%%%%%%%%%%%%%%%%%%%%%%%%%%%%%%%%%%%%%%%%%%

if ModelingMode==0
    % Values are all set to zero.
    JointTorqueLF=0;
elseif ModelingMode==1
    % Control based strategy. Values are based on difference in value
    % between the current state and desired state.
    % LF Joint Rotational Deltas
    DeltaLFPosition=LFPosition-TargetLFPosition;
    DeltaLFVelocity=LFVelocity-TargetLFVelocity;
    % Control Based Strategy
    JointTorqueLF=DeltaLFPosition*LFPCGain*GlobalPCGain-DeltaLFVelocity*LFVCGain*GlobalVCGain-DampeningGlobalGain*LFDampening*LFVelocity;
elseif ModelingMode==2
    % Forward Dynamics Based Strategy. Values are computed based on a
    % polynomial and a combination of dampening and position gained
    % factors.
    JointTorqueLF=Killswitch*GlobalGain*(LFConstant+LFTimeGain*Time-LFPositionGain*(LFPosition-LFPositionSetpoint)...
    -LFDampening*LFVelocity);
elseif ModelingMode==3
    JointTorqueLF=HexPolyInputFunction(LFInputA,LFInputB,LFInputC,LFInputD,LFInputE,LFInputF,LFInputG,Time)*Killswitch;
else
    %ZVCF Based Joint Torques. Values are pulled from model workspace and
    %held constant.
    JointTorqueLF=ZVCFLFTorque;
end

% %%%%%%%%%%%%%%%%%%%%%%%%%%%%%%%%%%%%%%%%%%%
% % Kinematic Input Selection and Calculation
% %%%%%%%%%%%%%%%%%%%%%%%%%%%%%%%%%%%%%%%%%%%

if KinematicMode==0
    % All kinematic values set to zero.
    LFPositionInput=0;
    LFVelocityInput=0;
    LFAccelerationInput=0;
elseif KinematicMode==1
    % 1st Order Acceleration, 2nd Order Velocity, 3rd Order Position Solution
    PTX=TargetLFPosition;       
    VTX=TargetLFVelocity;
    % Define Starting Position and Velocity
    PIX=LFStartPosition;
    VIX=LFStartVelocity;
    AX=3*((VTX+VIX)*TargetImpactTime-2*(PTX-PIX))/TargetImpactTime^3;         % Constant in position equation
    BX=-2*((VTX+2*VIX)*TargetImpactTime-3*(PTX-PIX))/TargetImpactTime^2;         % Constant in position equation
    CX=VIX;         % Starting Velocity at Time Zero
    DX=PIX;         % Starting Position at Time Zero
    % Equation for position as a function of time
    LFPositionInput=AX*Time^3/3+BX*Time^2/2+CX*Time+DX;
    LFVelocityInput=AX*Time^2+BX*Time+CX;
    LFAccelerationInput=2*AX*Time+BX;
elseif KinematicMode==2
    % 2nd Order Acceleration, 3rd Order Velocity, 4th Order Position Solution
    Tt=TargetImpactTime;
    t=Time;
    PoX=LFStartPosition;
    VoX=LFStartVelocity;
    PfX=TargetLFPosition;
    VfX=TargetLFVelocity;
    AoX=LFAo;
    LFPositionInput=PoX + VoX*t + (AoX*t^2)/2 - (t^3*(4*PoX - 4*PfX + Tt*VfX + 3*Tt*VoX + AoX*Tt^2))/Tt^3 + (t^4*(6*PoX - 6*PfX + 2*Tt*VfX + 4*Tt*VoX + AoX*Tt^2))/(2*Tt^4);
    LFVelocityInput=VoX + AoX*t - (3*t^2*(4*PoX - 4*PfX + Tt*VfX + 3*Tt*VoX + AoX*Tt^2))/Tt^3 + (2*t^3*(6*PoX - 6*PfX + 2*Tt*VfX + 4*Tt*VoX + AoX*Tt^2))/Tt^4;
    LFAccelerationInput=AoX + (6*t^2*(6*PoX - 6*PfX + 2*Tt*VfX + 4*Tt*VoX + AoX*Tt^2))/Tt^4 - (6*t*(4*PoX - 4*PfX + Tt*VfX + 3*Tt*VoX + AoX*Tt^2))/Tt^3;
else
    % 3rd Order Acceleration, 4th Order Velocity, 5th Order Position Solution
    Tt=TargetImpactTime;
    t=Time;
    PoX=LFStartPosition;
    VoX=LFStartVelocity;
    PfX=TargetLFPosition;
    VfX=TargetLFVelocity;
    AoX=LFAo;
    AfX=LFAf;
    LFPositionInput=PoX+VoX*t+(AoX*t^2)/2-(t^5*(12*PoX-12*PfX+6*Tt*VfX+6*Tt*VoX-AfX*Tt^2+AoX*Tt^2))/(2*Tt^5)-(t^3*(20*PoX-20*PfX+8*Tt*VfX+12*Tt*VoX-AfX*Tt^2+3*AoX*Tt^2))/(2*Tt^3)+(t^4*(30*PoX-30*PfX+14*Tt*VfX+16*Tt*VoX-2*AfX*Tt^2+3*AoX*Tt^2))/(2*Tt^4);
    LFVelocityInput=VoX+AoX*t-(5*t^4*(12*PoX-12*PfX+6*Tt*VfX+6*Tt*VoX-AfX*Tt^2+AoX*Tt^2))/(2*Tt^5)-(3*t^2*(20*PoX-20*PfX+8*Tt*VfX+12*Tt*VoX-AfX*Tt^2+3*AoX*Tt^2))/(2*Tt^3)+(2*t^3*(30*PoX-30*PfX+14*Tt*VfX+16*Tt*VoX-2*AfX*Tt^2+3*AoX*Tt^2))/Tt^4;
    LFAccelerationInput=AoX-(3*t*(20*PoX-20*PfX+8*Tt*VfX+12*Tt*VoX-AfX*Tt^2+3*AoX*Tt^2))/Tt^3-(10*t^3*(12*PoX-12*PfX+6*Tt*VfX+6*Tt*VoX-AfX*Tt^2+AoX*Tt^2))/Tt^5+(6*t^2*(30*PoX-30*PfX+14*Tt*VfX+16*Tt*VoX-2*AfX*Tt^2+3*AoX*Tt^2))/Tt^4;
end

% Calculate Higher Order Derivatives of the Position Outputs
LFJerk=gradient(LFAccelerationInput,t);
LFSnap=gradient(LFJerk,t);
LFCrackle=gradient(LFSnap,t);
LFPop=gradient(LFCrackle,t);
